simulink model "linsim2"  (R2022b)
settings: Solver=VariableStepAuto  StartTime=0.0  StopTime=20  FixedStep=1e-2  MaxStep=1e-2  RelTol=1e-4
values from neighbouring files (symbols this model uses):
  a = 1    [kalmf_rep.m]    (also in noise_01.m = 2)
  Q = 1    [O1sys0.m]    (also in kalmf_rep.m; noise_01.m; noise_02.m = eye(1))
undefined symbols (not defined in the file or in its folder): h
libraries: simulink x1
settings Model: Creator=hp_desktop  LastModifiedBy=hp_desktop

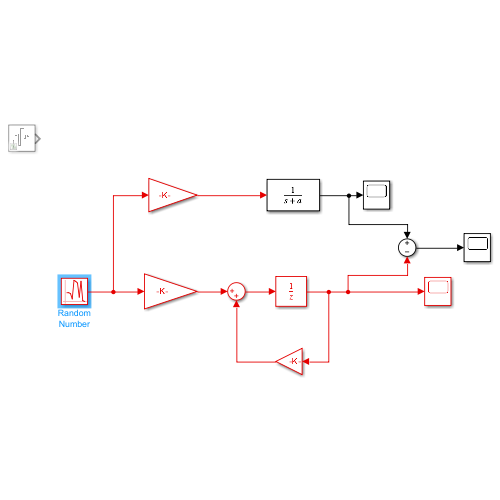
[thumbnail: Simulink's stored preview of the top-level diagram]
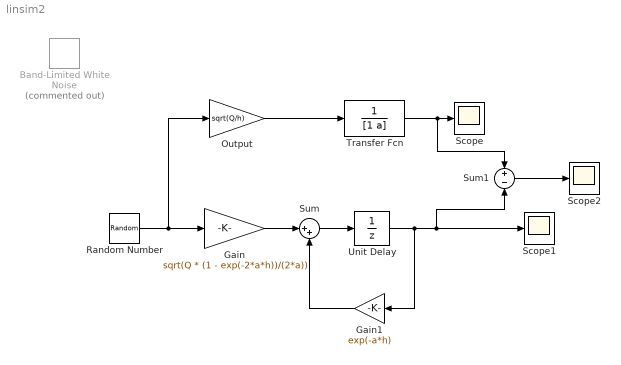
== system linsim2 ==
  Band-Limited White Noise : simulink/Sources/Band-Limited White Noise  Commented=on  Cov=1  Ts=h  seed=0
  Gain : Gain  Gain=sqrt(Q * (1 - exp(-2*a*h))/(2*a))
  Gain1 : Gain  Gain=exp(-a*h)
  Output : Gain  Gain=sqrt(Q/h)  SaturateOnIntegerOverflow=on  OutDataTypeStr=Inherit: Same as input  ParamDataTypeStr=Inherit: Same as input
  Random Number : RandomNumber  SampleTime=h
  Scope : Scope
  Scope1 : Scope
  Scope2 : Scope
  Sum : Sum  Inputs=|++
  Sum1 : Sum  Inputs=+-
  Transfer Fcn : TransferFcn  Denominator=[1 a]
  Unit Delay : UnitDelay  SampleTime=h  HasFrameUpgradeWarning=on
  wires:
  Transfer Fcn/1 -> Sum1/1, Scope/1
  Random Number/1 -> Output/1, Gain/1
  Unit Delay/1 -> Sum1/2, Scope1/1, Gain1/1
  Gain/1 -> Sum/1
  Sum/1 -> Unit Delay/1
  Gain1/1 -> Sum/2
  Output/1 -> Transfer Fcn/1
  Sum1/1 -> Scope2/1
